simulink library "sm_trackV_lib_terrain_contact_b9"  (R2026a)
settings: Solver=VariableStepAuto
undefined symbols (not defined in the file): B1, B2, B3, B4, B5, B6, B7, B8, L1, L2, L3, L4, L5, L6, L7, L8, L9, Road, S1, S2, Scene, X, Y, Z
libraries: $bdroot x20, sm_rollerV_lib_terrain_contact_belem x18, sm_excv_scene_lib x5, sm_lib x4, sm_trackV_lib_terrain_contact_elem x2
Description:
  | Copyright 2024-2026 The MathWorks, Inc.
settings Model: Creator=smiller  LastModifiedBy=smiller

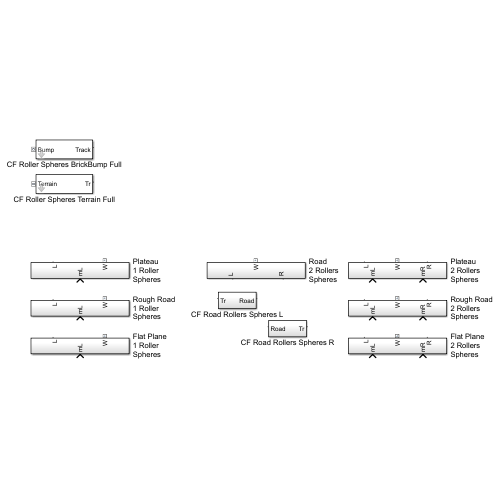
[thumbnail: Simulink's stored preview of the top-level diagram]
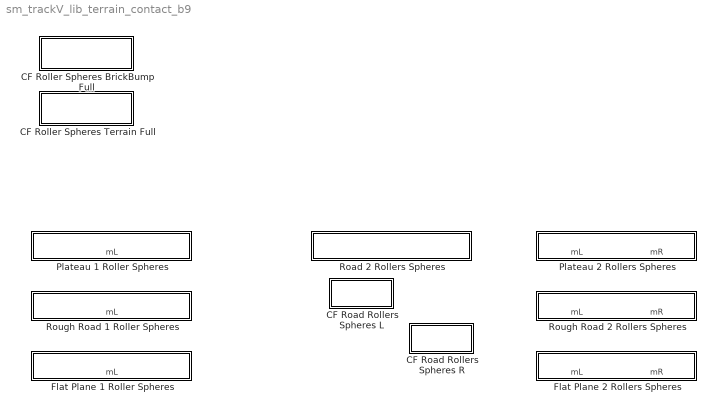
== system sm_trackV_lib_terrain_contact_b9 ==
  CF Road Rollers Spheres L : Subsystem
  CF Road Rollers Spheres R : Subsystem
  CF Roller Spheres BrickBump Full : Subsystem  mask(Contact Forces, Full Track to Bump){K_BrickBump=Scene.Contact.BrickBump.K, B_BrickBump=Scene.Contact.BrickBump.B, TW_BrickBump=Scene.Contact.BrickBump.TW}
      mask prompts: K_BrickBump "Normal Stiffness (N/m)"; B_BrickBump "Normal Damping (N/(m/s))"; TW_BrickBump "Normal Transition Width (m)"
      mask help: Models contact force between all spheres (two per rolling element) and a bump.
  CF Roller Spheres Terrain Full : Subsystem  mask(Contact Forces, All Rollers (Spheres) and Terrain)){K_Road=Scene.Contact.Terrain.K, B_Road=Scene.Contact.Terrain.B, TW_Road=Scene.Contact.Terrain.TW, F_dyn_Road=Scene.Contact.Terrain.mud, F_stat_Road=Scene.Contact.Terrain.mus, CV_Road=Scene.Contact.Terrain.CV}
      mask prompts: K_Road "Normal Stiffness (N/m)"; B_Road "Normal Damping (N/(m/s))"; TW_Road "Normal Transition Width (m)"; F_dyn_Road "Coefficient of Dynamic Friction"; F_stat_Road "Coefficient of Static Friction"; CV_Road "Critical Velocity (m/s)"
      mask help: Models contact force between all spheres (two per rolling element) and terrain.
  Flat Plane 1 Roller Spheres : Subsystem
  Flat Plane 2 Rollers Spheres : Subsystem
  Plateau 1 Roller Spheres : Subsystem
  Plateau 2 Rollers Spheres : Subsystem
  Road 2 Rollers Spheres : Subsystem
  Rough Road 1 Roller Spheres : Subsystem
  Rough Road 2 Rollers Spheres : Subsystem

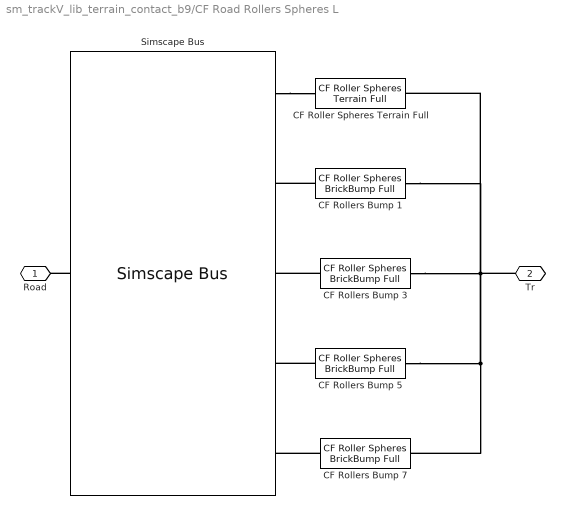
== system sm_trackV_lib_terrain_contact_b9/CF Road Rollers Spheres L ==
  CF Roller Spheres Terrain Full : $bdroot/CF Roller Spheres Terrain Full  K_Road=Scene.Contact.Terrain.K  B_Road=Scene.Contact.Terrain.B  TW_Road=Scene.Contact.Terrain.TW  F_dyn_Road=Scene.Contact.Terrain.mud  F_stat_Road=Scene.Contact.Terrain.mus  CV_Road=Scene.Contact.Terrain.CV
  CF Rollers Bump {1,3,5,7} (4 alike) : $bdroot/CF Roller Spheres BrickBump Full  K_BrickBump=Scene.Contact.BrickBump.K  B_BrickBump=Scene.Contact.BrickBump.B  TW_BrickBump=Scene.Contact.BrickBump.TW
  Simscape Bus : SimscapeBus  HierarchyStrings=Road;B1;B3;B5;B7  ConnectionType=Bus: CBO_Road8
  Road : PMIOPort  Side=Left
  Tr : PMIOPort  Port=2  Side=Right
  connections:
  CF Rollers Bump 3/LConn1 -- Simscape Bus/LConn3
  CF Rollers Bump 1/LConn1 -- Simscape Bus/LConn2
  Simscape Bus/LConn1 -- CF Roller Spheres Terrain Full/LConn1
  Simscape Bus/RConn1 -- Road/RConn1
  CF Rollers Bump 5/LConn1 -- Simscape Bus/LConn4
  CF Rollers Bump 7/LConn1 -- Simscape Bus/LConn5
  CF Rollers Bump 5/RConn1 -- CF Rollers Bump 7/RConn1 -- CF Rollers Bump 1/RConn1 -- CF Roller Spheres Terrain Full/RConn1 -- CF Rollers Bump 3/RConn1 -- Tr/RConn1

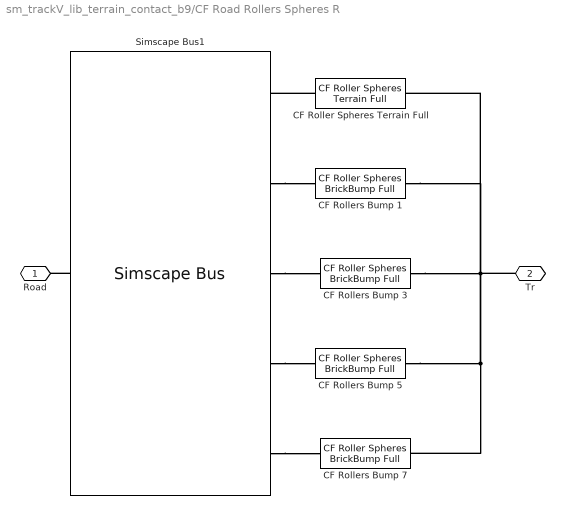
== system sm_trackV_lib_terrain_contact_b9/CF Road Rollers Spheres R ==
  CF Roller Spheres Terrain Full : $bdroot/CF Roller Spheres Terrain Full  K_Road=Scene.Contact.Terrain.K  B_Road=Scene.Contact.Terrain.B  TW_Road=Scene.Contact.Terrain.TW  F_dyn_Road=Scene.Contact.Terrain.mud  F_stat_Road=Scene.Contact.Terrain.mus  CV_Road=Scene.Contact.Terrain.CV
  CF Rollers Bump {1,3,5,7} (4 alike) : $bdroot/CF Roller Spheres BrickBump Full  K_BrickBump=Scene.Contact.BrickBump.K  B_BrickBump=Scene.Contact.BrickBump.B  TW_BrickBump=Scene.Contact.BrickBump.TW
  Simscape Bus1 : SimscapeBus  HierarchyStrings=Road;B2;B4;B6;B8  ConnectionType=Bus: CBO_Road8
  Road : PMIOPort  Side=Left
  Tr : PMIOPort  Port=2  Side=Right
  connections:
  CF Rollers Bump 5/RConn1 -- Tr/RConn1 -- CF Rollers Bump 3/RConn1 -- CF Rollers Bump 1/RConn1 -- CF Roller Spheres Terrain Full/RConn1 -- CF Rollers Bump 7/RConn1
  Simscape Bus1/LConn5 -- CF Rollers Bump 7/LConn1
  Simscape Bus1/LConn4 -- CF Rollers Bump 5/LConn1
  Simscape Bus1/RConn1 -- Road/RConn1
  CF Roller Spheres Terrain Full/LConn1 -- Simscape Bus1/LConn1
  Simscape Bus1/LConn2 -- CF Rollers Bump 1/LConn1
  Simscape Bus1/LConn3 -- CF Rollers Bump 3/LConn1

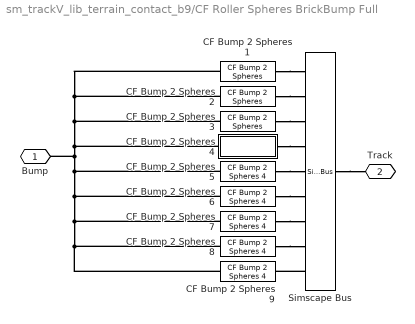
== system sm_trackV_lib_terrain_contact_b9/CF Roller Spheres BrickBump Full ==
  CF Bump 2 Spheres 1 : sm_rollerV_lib_terrain_contact_belem/CF Bump 2 Spheres  K_BrickBump=K_BrickBump  B_BrickBump=B_BrickBump  TW_BrickBump=TW_BrickBump  CoefficientOfDynamicFriction=Scene.Contact.Terrain.mud  CoefficientOfStaticFriction=Scene.Contact.Terrain.mus  FrictionalCriticalVelocity=Scene.Contact.Terrain.CV
  CF Bump 2 Spheres 2 : sm_rollerV_lib_terrain_contact_belem/CF Bump 2 Spheres  K_BrickBump=K_BrickBump  B_BrickBump=B_BrickBump  TW_BrickBump=TW_BrickBump  CoefficientOfDynamicFriction=Scene.Contact.Terrain.mud  CoefficientOfStaticFriction=Scene.Contact.Terrain.mus  FrictionalCriticalVelocity=Scene.Contact.Terrain.CV
  CF Bump 2 Spheres 3 : sm_rollerV_lib_terrain_contact_belem/CF Bump 2 Spheres  K_BrickBump=K_BrickBump  B_BrickBump=B_BrickBump  TW_BrickBump=TW_BrickBump  CoefficientOfDynamicFriction=Scene.Contact.Terrain.mud  CoefficientOfStaticFriction=Scene.Contact.Terrain.mus  FrictionalCriticalVelocity=Scene.Contact.Terrain.CV
  CF Bump 2 Spheres 4 : Subsystem  mask{K_BrickBump=K_BrickBump, B_BrickBump=B_BrickBump, TW_BrickBump=TW_BrickBump}
      mask prompts: K_BrickBump "Normal Stiffness (N/m)"; B_BrickBump "Normal Damping (N/(m/s))"; TW_BrickBump "Normal Transition Width (m)"
      mask TypeOptions K_BrickBump: CF Bump Roller Sphere 1 /NormalStiffness | CF Bump Roller Sphere 2/NormalStiffness
      mask TypeOptions B_BrickBump: CF Bump Roller Sphere 1 /NormalDamping | CF Bump Roller Sphere 2/NormalDamping
      mask TypeOptions TW_BrickBump: CF Bump Roller Sphere 1 /NormalTransitionRegionWidth | CF Bump Roller Sphere 2/NormalTransitionRegionWidth
  CF Bump 2 Spheres {5..9} (5 alike) : $bdroot/CF Roller Spheres BrickBump Full/CF Bump 2 Spheres 4  K_BrickBump=K_BrickBump  B_BrickBump=B_BrickBump  TW_BrickBump=TW_BrickBump
  Simscape Bus : SimscapeBus  HierarchyStrings=L1;L2;L3;L4;L5;L6;L7;L8;L9
  Bump : PMIOPort  Side=Left
  Track : PMIOPort  Port=2  Side=Right
  connections:
  CF Bump 2 Spheres 6/LConn1 -- CF Bump 2 Spheres 5/LConn1 -- CF Bump 2 Spheres 4/LConn1 -- CF Bump 2 Spheres 3/LConn1 -- CF Bump 2 Spheres 2/LConn1 -- CF Bump 2 Spheres 1/LConn1 -- Bump/RConn1 -- CF Bump 2 Spheres 7/LConn1 -- CF Bump 2 Spheres 8/LConn1 -- CF Bump 2 Spheres 9/LConn1
  Simscape Bus/RConn1 -- Track/RConn1
  CF Bump 2 Spheres 4/RConn1 -- Simscape Bus/LConn4
  CF Bump 2 Spheres 2/RConn1 -- Simscape Bus/LConn2
  CF Bump 2 Spheres 8/RConn1 -- Simscape Bus/LConn8
  CF Bump 2 Spheres 7/RConn1 -- Simscape Bus/LConn7
  CF Bump 2 Spheres 6/RConn1 -- Simscape Bus/LConn6
  CF Bump 2 Spheres 3/RConn1 -- Simscape Bus/LConn3
  CF Bump 2 Spheres 5/RConn1 -- Simscape Bus/LConn5
  Simscape Bus/LConn9 -- CF Bump 2 Spheres 9/RConn1
  CF Bump 2 Spheres 1/RConn1 -- Simscape Bus/LConn1

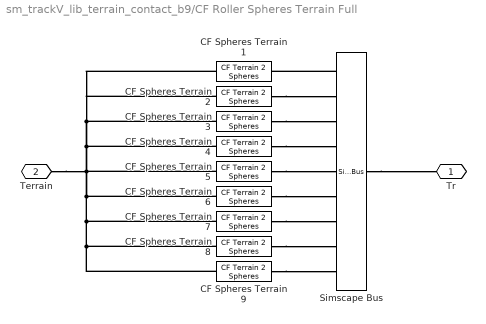
== system sm_trackV_lib_terrain_contact_b9/CF Roller Spheres Terrain Full ==
  CF Spheres Terrain {1..9} (9 alike) : sm_rollerV_lib_terrain_contact_belem/CF Terrain 2 Spheres  NormalStiffness=K_Road  NormalDamping=B_Road  NormalTransitionRegionWidth=TW_Road  CoefficientOfDynamicFriction=F_dyn_Road  CoefficientOfStaticFriction=F_stat_Road  FrictionalCriticalVelocity=CV_Road
  Simscape Bus : SimscapeBus  HierarchyStrings=L1;L2;L3;L4;L5;L6;L7;L8;L9
  Tr : PMIOPort  Side=Right
  Terrain : PMIOPort  Port=2  Side=Left
  connections:
  CF Spheres Terrain 9/RConn1 -- Simscape Bus/LConn9
  CF Spheres Terrain 8/RConn1 -- Simscape Bus/LConn8
  CF Spheres Terrain 7/RConn1 -- Simscape Bus/LConn7
  CF Spheres Terrain 6/RConn1 -- Simscape Bus/LConn6
  CF Spheres Terrain 5/RConn1 -- Simscape Bus/LConn5
  CF Spheres Terrain 4/RConn1 -- Simscape Bus/LConn4
  CF Spheres Terrain 3/RConn1 -- Simscape Bus/LConn3
  CF Spheres Terrain 2/RConn1 -- Simscape Bus/LConn2
  Simscape Bus/LConn1 -- CF Spheres Terrain 1/RConn1
  Simscape Bus/RConn1 -- Tr/RConn1
  CF Spheres Terrain 9/LConn1 -- CF Spheres Terrain 8/LConn1 -- CF Spheres Terrain 7/LConn1 -- CF Spheres Terrain 6/LConn1 -- CF Spheres Terrain 5/LConn1 -- Terrain/RConn1 -- CF Spheres Terrain 4/LConn1 -- CF Spheres Terrain 3/LConn1 -- CF Spheres Terrain 2/LConn1 -- CF Spheres Terrain 1/LConn1

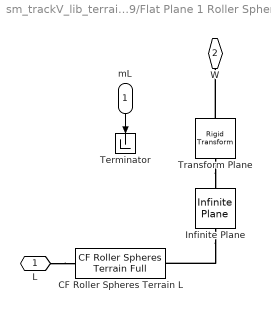
== system sm_trackV_lib_terrain_contact_b9/Flat Plane 1 Roller Spheres ==
  mL : Inport
  CF Roller Spheres Terrain L : $bdroot/CF Roller Spheres Terrain Full  K_Road=Scene.Contact.Spheres.Terrain.K  B_Road=Scene.Contact.Spheres.Terrain.B  TW_Road=Scene.Contact.Spheres.Terrain.TW  F_dyn_Road=Scene.Contact.Spheres.Terrain.mud  F_stat_Road=Scene.Contact.Spheres.Terrain.mus  CV_Road=Scene.Contact.Spheres.Terrain.CV
  Infinite Plane : sm_lib/Curves and Surfaces/Infinite Plane  GraphicType=Rectangle  GraphicPlaneWidth=Scene.Plane.l  GraphicPlaneWidthUnits=m  GraphicPlaneHeight=Scene.Plane.w  GraphicPlaneHeightUnits=m  GraphicVisPropType=SimpleVisualProperties  GraphicDiffuseColor=[0.5 0.5 0.5]  GraphicOpacity=0.25  GraphicSpecularColor=[0.5 0.5 0.5 1.0]  GraphicAmbientColor=[0.15 0.15 0.15 1.0]  GraphicEmissiveColor=[0.0 0.0 0.0 1.0]  GraphicShininess=75
  Terminator : Terminator
  Transform Plane : sm_lib/Frames and Transforms/Rigid Transform  RotationMethod=None  FollAlignAxisA=+X  BaseAlignAxisA=+Y  FollAlignAxisB=+Y  BaseAlignAxisB=+Z  RotationStandardAxis=+Z  RotationAngle=0.0  RotationAngleUnits=deg  RotationArbitraryAxis=[0 0 1]  RotationSequenceAxes=FollowerAxes  RotationSequence=XYX  RotationSequenceAngles=[0 0 0]  RotationSequenceAnglesUnits=deg  RotationMatrix=[1 0 0; 0 1 0; 0 0 1]  Quaternion=[1 0 0 0]  TranslationMethod=Cartesian  TranslationCartesianOffset=Scene.Plane.offset  TranslationCartesianOffsetUnits=m  TranslationStandardAxis=+Z  TranslationStandardOffset=0  TranslationStandardOffsetUnits=m  TranslationROffset=0  TranslationROffsetUnits=m  TranslationThetaOffset=0  TranslationThetaOffsetUnits=deg  TranslationZOffset=0  TranslationZOffsetUnits=m
  L : PMIOPort  Side=Right
  W : PMIOPort  Port=2  Side=Right
  wires:
  mL/1 -> Terminator/1
  connections:
  Transform Plane/LConn1 -- W/RConn1
  Transform Plane/RConn1 -- Infinite Plane/LConn1
  L/RConn1 -- CF Roller Spheres Terrain L/RConn1
  Infinite Plane/RConn1 -- CF Roller Spheres Terrain L/LConn1

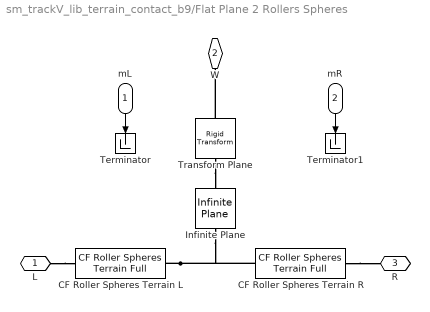
== system sm_trackV_lib_terrain_contact_b9/Flat Plane 2 Rollers Spheres ==
  mL : Inport
  mR : Inport  Port=2
  CF Roller Spheres Terrain L : $bdroot/CF Roller Spheres Terrain Full  K_Road=Scene.Contact.Spheres.Terrain.K  B_Road=Scene.Contact.Spheres.Terrain.B  TW_Road=Scene.Contact.Spheres.Terrain.TW  F_dyn_Road=Scene.Contact.Spheres.Terrain.mud  F_stat_Road=Scene.Contact.Spheres.Terrain.mus  CV_Road=Scene.Contact.Spheres.Terrain.CV
  CF Roller Spheres Terrain R : $bdroot/CF Roller Spheres Terrain Full  K_Road=Scene.Contact.Spheres.Terrain.K  B_Road=Scene.Contact.Spheres.Terrain.B  TW_Road=Scene.Contact.Spheres.Terrain.TW  F_dyn_Road=Scene.Contact.Spheres.Terrain.mud  F_stat_Road=Scene.Contact.Spheres.Terrain.mus  CV_Road=Scene.Contact.Spheres.Terrain.CV
  Infinite Plane : sm_lib/Curves and Surfaces/Infinite Plane  GraphicType=Rectangle  GraphicPlaneWidth=Scene.Plane.l  GraphicPlaneWidthUnits=m  GraphicPlaneHeight=Scene.Plane.w  GraphicPlaneHeightUnits=m  GraphicVisPropType=SimpleVisualProperties  GraphicDiffuseColor=[0.5 0.5 0.5]  GraphicOpacity=0.25  GraphicSpecularColor=[0.5 0.5 0.5 1.0]  GraphicAmbientColor=[0.15 0.15 0.15 1.0]  GraphicEmissiveColor=[0.0 0.0 0.0 1.0]  GraphicShininess=75
  Terminator : Terminator
  Terminator1 : Terminator
  Transform Plane : sm_lib/Frames and Transforms/Rigid Transform  RotationMethod=None  FollAlignAxisA=+X  BaseAlignAxisA=+Y  FollAlignAxisB=+Y  BaseAlignAxisB=+Z  RotationStandardAxis=+Z  RotationAngle=0.0  RotationAngleUnits=deg  RotationArbitraryAxis=[0 0 1]  RotationSequenceAxes=FollowerAxes  RotationSequence=XYX  RotationSequenceAngles=[0 0 0]  RotationSequenceAnglesUnits=deg  RotationMatrix=[1 0 0; 0 1 0; 0 0 1]  Quaternion=[1 0 0 0]  TranslationMethod=Cartesian  TranslationCartesianOffset=Scene.Plane.offset  TranslationCartesianOffsetUnits=m  TranslationStandardAxis=+Z  TranslationStandardOffset=0  TranslationStandardOffsetUnits=m  TranslationROffset=0  TranslationROffsetUnits=m  TranslationThetaOffset=0  TranslationThetaOffsetUnits=deg  TranslationZOffset=0  TranslationZOffsetUnits=m
  L : PMIOPort  Side=Right
  W : PMIOPort  Port=2  Side=Right
  R : PMIOPort  Port=3  Side=Right
  wires:
  mR/1 -> Terminator1/1
  mL/1 -> Terminator/1
  connections:
  CF Roller Spheres Terrain L/LConn1 -- Infinite Plane/RConn1 -- CF Roller Spheres Terrain R/LConn1
  CF Roller Spheres Terrain R/RConn1 -- R/RConn1
  L/RConn1 -- CF Roller Spheres Terrain L/RConn1
  Transform Plane/RConn1 -- Infinite Plane/LConn1
  Transform Plane/LConn1 -- W/RConn1

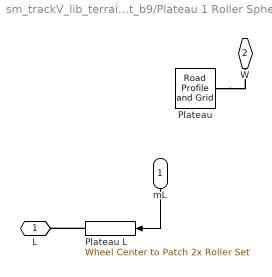
== system sm_trackV_lib_terrain_contact_b9/Plateau 1 Roller Spheres ==
  mL : Inport
  Plateau : sm_excv_scene_lib/Road Profile and Grid  VariantControl=Plateau  RDF_Polyline=Scene.Plateau  grid_z_offset=0  grid_x=Scene.Grid.length*0.7  grid_y=Scene.Grid.width*0.01  grid_z=Scene.Grid.depth  grid_line_width=Scene.Grid.linewidth  grid_num_sq_x=Scene.Grid.numsquaresx*0.7  grid_num_sq_y=Scene.Grid.numsquaresy*0.01  plane_clr=Scene.Grid.planecolor  grid_clr=Scene.Grid.linecolor  grid_opc=1
      settings: LibrarySourceBlock=sm_excv_uneven_road_lib/Plateau
  Plateau L : sm_rollerV_lib_terrain_contact_belem/Wheel Center to Patch 2x Roller Set  road_pz_x=Scene.Plateau.Road.pzLUT.px  road_pz_z=Scene.Plateau.Road.pzLUT.pz(:,1)  road_qy_x=Scene.Plateau.Road.qyLUT.px  road_qy_qy=Scene.Plateau.Road.qyLUT.qy(:,1)  tfilter=0.01  NormalStiffness=Scene.Contact.Terrain.K  NormalDamping=Scene.Contact.Terrain.B  NormalTransitionRegionWidth=Scene.Contact.Terrain.TW  CoefficientOfDynamicFriction=Scene.Contact.Terrain.mud  CoefficientOfStaticFriction=Scene.Contact.Terrain.mus  FrictionalCriticalVelocity=Scene.Contact.Terrain.CV  patch_x=Scene.Patch.w  patch_y=Scene.Patch.l  patch_clr=Scene.Patch.clr  patch_opc=Scene.Patch.opc
      settings: LibrarySourceBlock=sm_excv_uneven_road_lib/Rollers Rough Road1
  L : PMIOPort  Side=Right
  W : PMIOPort  Port=2  Side=Right
  wires:
  mL/1 -> Plateau L/1
  connections:
  Plateau/RConn1 -- W/RConn1
  Plateau L/RConn1 -- L/RConn1

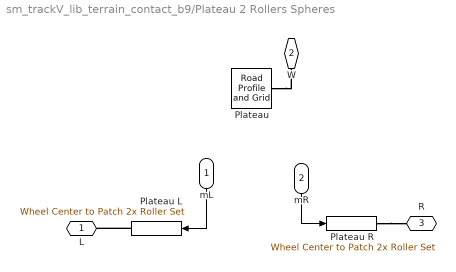
== system sm_trackV_lib_terrain_contact_b9/Plateau 2 Rollers Spheres ==
  mL : Inport
  mR : Inport  Port=2
  Plateau : sm_excv_scene_lib/Road Profile and Grid  VariantControl=Plateau  RDF_Polyline=Scene.Plateau  grid_z_offset=0  grid_x=Scene.Grid.length*0.7  grid_y=Scene.Grid.width*0.01  grid_z=Scene.Grid.depth  grid_line_width=Scene.Grid.linewidth  grid_num_sq_x=Scene.Grid.numsquaresx*0.7  grid_num_sq_y=Scene.Grid.numsquaresy*0.01  plane_clr=Scene.Grid.planecolor  grid_clr=Scene.Grid.linecolor  grid_opc=1
      settings: LibrarySourceBlock=sm_excv_uneven_road_lib/Plateau
  Plateau L : sm_rollerV_lib_terrain_contact_belem/Wheel Center to Patch 2x Roller Set  road_pz_x=Scene.Plateau.Road.pzLUT.px  road_pz_z=Scene.Plateau.Road.pzLUT.pz(:,1)  road_qy_x=Scene.Plateau.Road.qyLUT.px  road_qy_qy=Scene.Plateau.Road.qyLUT.qy(:,1)  tfilter=0.01  NormalStiffness=Scene.Contact.Terrain.K  NormalDamping=Scene.Contact.Terrain.B  NormalTransitionRegionWidth=Scene.Contact.Terrain.TW  CoefficientOfDynamicFriction=Scene.Contact.Terrain.mud  CoefficientOfStaticFriction=Scene.Contact.Terrain.mus  FrictionalCriticalVelocity=Scene.Contact.Terrain.CV  patch_x=Scene.Patch.w  patch_y=Scene.Patch.l  patch_clr=Scene.Patch.clr  patch_opc=Scene.Patch.opc
      settings: LibrarySourceBlock=sm_excv_uneven_road_lib/Rollers Rough Road1
  Plateau R : sm_rollerV_lib_terrain_contact_belem/Wheel Center to Patch 2x Roller Set  road_pz_x=Scene.Plateau.Road.pzLUT.px  road_pz_z=Scene.Plateau.Road.pzLUT.pz(:,2)  road_qy_x=Scene.Plateau.Road.qyLUT.px  road_qy_qy=Scene.Plateau.Road.qyLUT.qy(:,2)  tfilter=0.01  NormalStiffness=Scene.Contact.Terrain.K  NormalDamping=Scene.Contact.Terrain.B  NormalTransitionRegionWidth=Scene.Contact.Terrain.TW  CoefficientOfDynamicFriction=Scene.Contact.Terrain.mud  CoefficientOfStaticFriction=Scene.Contact.Terrain.mus  FrictionalCriticalVelocity=Scene.Contact.Terrain.CV  patch_x=Scene.Patch.w  patch_y=Scene.Patch.l  patch_clr=Scene.Patch.clr  patch_opc=Scene.Patch.opc
      settings: LibrarySourceBlock=sm_excv_uneven_road_lib/Rollers Rough Road1
  L : PMIOPort  Side=Right
  W : PMIOPort  Port=2  Side=Right
  R : PMIOPort  Port=3  Side=Right
  wires:
  mR/1 -> Plateau R/1
  mL/1 -> Plateau L/1
  connections:
  Plateau L/RConn1 -- L/RConn1
  Plateau/RConn1 -- W/RConn1
  Plateau R/RConn1 -- R/RConn1

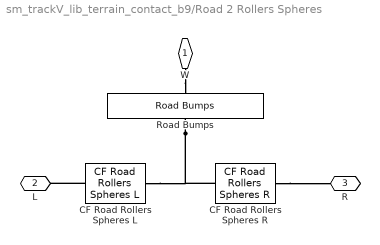
== system sm_trackV_lib_terrain_contact_b9/Road 2 Rollers Spheres ==
  CF Road Rollers Spheres L : $bdroot/CF Road Rollers Spheres L  SystemSampleTime=-1  VariantActivationTime=update diagram  EmptyChoice=off  PassThrough=off  PassThroughVariantControl=(default)  EmptyChoiceVariantControl=(default)  AllowFlexibleInterface=on  Latency=0  AutoFrameSizeCalculation=off
  CF Road Rollers Spheres R : $bdroot/CF Road Rollers Spheres R  SystemSampleTime=-1  VariantActivationTime=update diagram  EmptyChoice=off  PassThrough=off  PassThroughVariantControl=(default)  EmptyChoiceVariantControl=(default)  AllowFlexibleInterface=on  Latency=0  AutoFrameSizeCalculation=off
  Road Bumps : sm_excv_scene_lib/Road Bumps  road_x=Scene.Road.len  road_y=Scene.Road.wid  road_z=Scene.Road.hgt  bump_x=Scene.Road.Bump.len  bump_y=Scene.Road.Bump.wid  bump_z=Scene.Road.Bump.hgt  bloc_y=Scene.Road.Bump.offsety  bloc_z=Scene.Road.Bump.offsetz  bump_x0=Scene.Road.Bump.startx  bloc_dx=Scene.Road.Bump.deltax
  W : PMIOPort  Side=Right
  L : PMIOPort  Port=2  Side=Left
  R : PMIOPort  Port=3  Side=Left
  connections:
  CF Road Rollers Spheres L/RConn1 -- L/RConn1
  Road Bumps/LConn1 -- CF Road Rollers Spheres R/LConn1 -- CF Road Rollers Spheres L/LConn1
  W/RConn1 -- Road Bumps/RConn1
  CF Road Rollers Spheres R/RConn1 -- R/RConn1

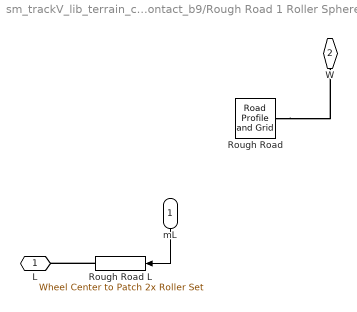
== system sm_trackV_lib_terrain_contact_b9/Rough Road 1 Roller Spheres ==
  mL : Inport
  Rough Road : sm_excv_scene_lib/Road Profile and Grid  VariantControl=Plateau  RDF_Polyline=Scene.Rough_Road  grid_z_offset=-0.2  grid_x=Scene.Grid.length*0.5  grid_y=Scene.Grid.width*0.01  grid_z=Scene.Grid.depth  grid_line_width=Scene.Grid.linewidth  grid_num_sq_x=Scene.Grid.numsquaresx*0.5  grid_num_sq_y=Scene.Grid.numsquaresy*0.01  plane_clr=Scene.Grid.linecolor  grid_clr=Scene.Grid.planecolor  grid_opc=1
  Rough Road L : sm_rollerV_lib_terrain_contact_belem/Wheel Center to Patch 2x Roller Set  road_pz_x=Scene.Rough_Road.Road.pzLUT.px  road_pz_z=Scene.Rough_Road.Road.pzLUT.pz(:,1)  road_qy_x=Scene.Rough_Road.Road.qyLUT.px  road_qy_qy=Scene.Rough_Road.Road.qyLUT.qy(:,1)  tfilter=0.01  NormalStiffness=Scene.Contact.Terrain.K  NormalDamping=Scene.Contact.Terrain.B  NormalTransitionRegionWidth=Scene.Contact.Terrain.TW  CoefficientOfDynamicFriction=Scene.Contact.Terrain.mud  CoefficientOfStaticFriction=Scene.Contact.Terrain.mus  FrictionalCriticalVelocity=Scene.Contact.Terrain.CV  patch_x=Scene.Patch.w  patch_y=Scene.Patch.l  patch_clr=Scene.Patch.clr  patch_opc=Scene.Patch.opc
      settings: LibrarySourceBlock=sm_excv_uneven_road_lib/Rollers Rough Road1
  L : PMIOPort  Side=Right
  W : PMIOPort  Port=2  Side=Right
  wires:
  mL/1 -> Rough Road L/1
  connections:
  Rough Road L/RConn1 -- L/RConn1
  Rough Road/RConn1 -- W/RConn1

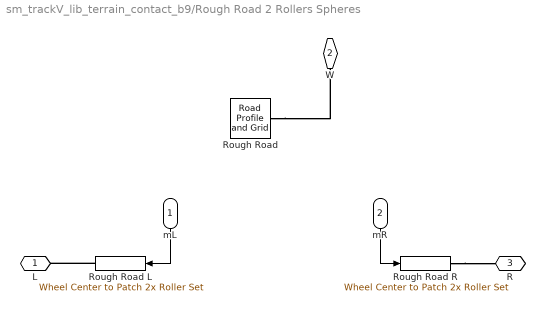
== system sm_trackV_lib_terrain_contact_b9/Rough Road 2 Rollers Spheres ==
  mL : Inport
  mR : Inport  Port=2
  Rough Road : sm_excv_scene_lib/Road Profile and Grid  VariantControl=Plateau  RDF_Polyline=Scene.Rough_Road  grid_z_offset=-0.2  grid_x=Scene.Grid.length*0.5  grid_y=Scene.Grid.width*0.01  grid_z=Scene.Grid.depth  grid_line_width=Scene.Grid.linewidth  grid_num_sq_x=Scene.Grid.numsquaresx*0.5  grid_num_sq_y=Scene.Grid.numsquaresy*0.01  plane_clr=Scene.Grid.linecolor  grid_clr=Scene.Grid.planecolor  grid_opc=1
  Rough Road L : sm_rollerV_lib_terrain_contact_belem/Wheel Center to Patch 2x Roller Set  road_pz_x=Scene.Rough_Road.Road.pzLUT.px  road_pz_z=Scene.Rough_Road.Road.pzLUT.pz(:,1)  road_qy_x=Scene.Rough_Road.Road.qyLUT.px  road_qy_qy=Scene.Rough_Road.Road.qyLUT.qy(:,1)  tfilter=0.01  NormalStiffness=Scene.Contact.Terrain.K  NormalDamping=Scene.Contact.Terrain.B  NormalTransitionRegionWidth=Scene.Contact.Terrain.TW  CoefficientOfDynamicFriction=Scene.Contact.Terrain.mud  CoefficientOfStaticFriction=Scene.Contact.Terrain.mus  FrictionalCriticalVelocity=Scene.Contact.Terrain.CV  patch_x=Scene.Patch.w  patch_y=Scene.Patch.l  patch_clr=Scene.Patch.clr  patch_opc=Scene.Patch.opc
      settings: LibrarySourceBlock=sm_excv_uneven_road_lib/Rollers Rough Road1
  Rough Road R : sm_rollerV_lib_terrain_contact_belem/Wheel Center to Patch 2x Roller Set  road_pz_x=Scene.Rough_Road.Road.pzLUT.px  road_pz_z=Scene.Rough_Road.Road.pzLUT.pz(:,2)  road_qy_x=Scene.Rough_Road.Road.qyLUT.px  road_qy_qy=Scene.Rough_Road.Road.qyLUT.qy(:,2)  tfilter=0.01  NormalStiffness=Scene.Contact.Terrain.K  NormalDamping=Scene.Contact.Terrain.B  NormalTransitionRegionWidth=Scene.Contact.Terrain.TW  CoefficientOfDynamicFriction=Scene.Contact.Terrain.mud  CoefficientOfStaticFriction=Scene.Contact.Terrain.mus  FrictionalCriticalVelocity=Scene.Contact.Terrain.CV  patch_x=Scene.Patch.w  patch_y=Scene.Patch.l  patch_clr=Scene.Patch.clr  patch_opc=Scene.Patch.opc
      settings: LibrarySourceBlock=sm_excv_uneven_road_lib/Rollers Rough Road1
  L : PMIOPort  Side=Right
  W : PMIOPort  Port=2  Side=Right
  R : PMIOPort  Port=3  Side=Right
  wires:
  mL/1 -> Rough Road L/1
  mR/1 -> Rough Road R/1
  connections:
  Rough Road R/RConn1 -- R/RConn1
  Rough Road/RConn1 -- W/RConn1
  Rough Road L/RConn1 -- L/RConn1

== system sm_trackV_lib_terrain_contact_b9/CF Roller Spheres BrickBump Full/CF Bump 2 Spheres 4 ==
  "CF Bump Roller Sphere 1 " : sm_trackV_lib_terrain_contact_elem/CF Track BrickBump  NormalStiffness=K_BrickBump  NormalDamping=B_BrickBump  NormalTransitionRegionWidth=TW_BrickBump
  CF Bump Roller Sphere 2 : sm_trackV_lib_terrain_contact_elem/CF Track BrickBump  NormalStiffness=K_BrickBump  NormalDamping=B_BrickBump  NormalTransitionRegionWidth=TW_BrickBump
  Simscape Bus1 : SimscapeBus  HierarchyStrings=S1;S2
  Terrain : PMIOPort  Side=Left
  R : PMIOPort  Port=2  Side=Right
  connections:
  Simscape Bus1/RConn1 -- R/RConn1
  CF Bump Roller Sphere 2/RConn1 -- Simscape Bus1/LConn2
  "CF Bump Roller Sphere 1 "/LConn1 -- Terrain/RConn1 -- CF Bump Roller Sphere 2/LConn1
  "CF Bump Roller Sphere 1 "/RConn1 -- Simscape Bus1/LConn1
